simulink model "InductionMotorDrive"  (R2016a)
settings: Solver=FixedStepAuto  SolverMode=SingleTasking  StartTime=0.0  StopTime=5  FixedStep=1/400000  RelTol=1e-3
undefined symbols (not defined in the file): rad, s
libraries: powerlib x23, simulink x3, aerolibconvert2 x1, powerlib_meascontrol x1, electricdrivelib x1
settings Model: Creator=mrsmash  LastModifiedBy=mrsmash
settings SimscapeCC: SimscapeLogType=local  SimscapeLogName=simlog_Induction  SimscapeLogDataHistory=5000000

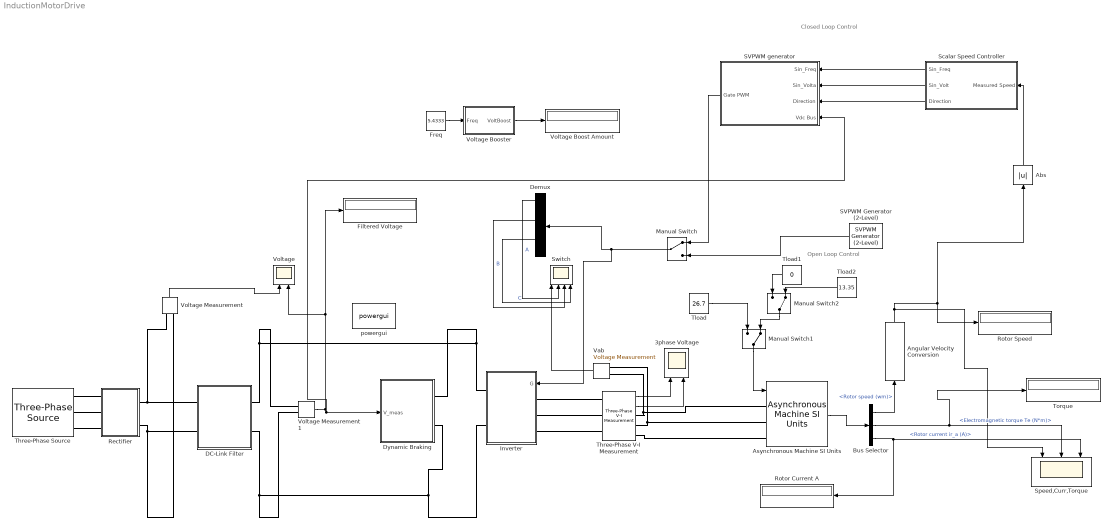
== system InductionMotorDrive ==
  note: Closed Loop Control
  note: Open Loop Control
  3phase Voltage : Scope  NumInputPorts=2
  Abs : Abs
  Angular Velocity Conversion : aerolibconvert2/Angular Velocity Conversion  IU=rad/s  OU=rpm
  Asynchronous Machine SI Units : powerlib/Machines/Asynchronous Machine SI Units  RotorType=Squirrel-cage  PresetModel=No  MechanicalLoad=Torque Tm  ShowDetailedParameters=on  ReferenceFrame=Rotor  Units=SI  MeasurementBus=off  NominalParameters=[4000 400 50]  Stator=[1.405 0.005839]  Rotor=[1.395 0.005839]  Cage1=[0.4155 0.002066]  Cage2=[0.4168 0.0003495]  Lm=0.1722  Mechanical=[0.04 0.002985 2]  PolePairs=2  InitialConditions=[1 0 0 0 0 0 0 0]  SimulateSaturation=off  Saturation=[14.03593122, 27.81365428, 53.79336849, 72.68890987, 97.98006896, 148.6815601, 215.7428561, 302.9841135, 428.7778367 ; 230, 322, 414, 460, 506, 552, 598, 644, 690]  LoadFlowParameters=1492000  TsPowergui=0  TsBlock=-1  IterativeModel=Trapezoidal non iterative  IterativeDiscreteModel=Trapezoidal non iterative  Pmec=1.492e+006
  Bus Selector : BusSelector  OutputSignals=Mechanical.Rotor speed (wm),Mechanical.Electromagnetic torque Te (N*m),Rotor measurements.Rotor current ir_a (A)
  DC-Link Filter : Subsystem
  Demux : Demux  Outputs=6
  Dynamic Braking : Subsystem
  Filtered Voltage : Display
  Freq : Constant  Value=5.4333
  Inverter : Subsystem
  Manual Switch : ManualSwitch
  Manual Switch1 : ManualSwitch  CurrentSetting=0
  Manual Switch2 : ManualSwitch  CurrentSetting=0
  Rectifier : Subsystem
  Rotor Current A : Display
  Rotor Speed : Display
  SVPWM Generator (2-Level) : powerlib_meascontrol/Pulse & Signal Generators/SVPWM Generator (2-Level)  InputType=Internally generated  SwitchingPattern=Pattern #2  Fc=10e3  ParUref=[0.1072985 0 5.43]  Ts=0
  SVPWM generator : Subsystem
  Scalar Speed Controller : Subsystem
  Speed,Curr,Torque : Scope  NumInputPorts=3
  Switch : Scope  NumInputPorts=4
  Three-Phase V-I Measurement : powerlib/Measurements/Three-Phase V-I Measurement  VoltageMeasurement=phase-to-ground  SetLabelV=off  LabelV=Vabc  Vpu=off  VpuLL=off  CurrentMeasurement=yes  SetLabelI=off  LabelI=Iabc  Ipu=off  Pbase=100e6  Vbase=500e3  OutputType=Complex  PhasorSimulation=off  PSBequivalent=0
  Three-Phase Source : powerlib/Electrical Sources/Three-Phase Source  InternalConnection=Yg  VoltagePhases=on  Voltage=25e3  PhaseAngle=0  Voltage_phases=[690 690 690]/sqrt(3)  PhaseAngles_phases=[0 -120 +120]  Frequency=50  NonIdealSource=off  SpecifyImpedance=off  Resistance=0.8929  Inductance=16.58e-3  ShortCircuitLevel=100e6  BaseVoltage=25e3  XRratio=7  BusType=swing  Pref=10e3  Qref=0  Prefabc=[10e3, 10e3, 10e3]  Qrefabc=[0, 0, 0]  Qmin=-inf  Qmax=inf
  Tload : Constant  Value=26.7
  Tload1 : Constant  Value=0
  Tload2 : Constant  Value=13.35
  Torque : Display
  Vab : powerlib/Measurements/Voltage Measurement  PhasorSimulation=off  OutputType=Complex  PSBequivalent=0
  Voltage : Scope  NumInputPorts=2
  Voltage Boost Amount : Display
  Voltage Booster : Subsystem
  Voltage Measurement : powerlib/Measurements/Voltage Measurement  PhasorSimulation=off  OutputType=Complex  PSBequivalent=0
  Voltage Measurement1 : powerlib/Measurements/Voltage Measurement  PhasorSimulation=off  OutputType=Complex  PSBequivalent=0
  powergui : powerlib/powergui  Priority=1  SimulationMode=Discrete  SolverType=Tustin/Backward Euler (TBE)  SampleTime=1/400000  frequency=60  SPID=on  DisableSnubberDevices=on  DisableRonSwitches=off  DisableVfSwitches=off  SwTol=0  DisplayEquations=off  Interpol=off  ExternalGateDelay=off  methode=off  Ts=10  FunctionMessages=off  echomessages=off  HookPort=off  EnableUseOfTLC=off  x0status=blocks  frequencyindice=50  Pbase=100e6  ErrMax=1e-4  Iterations=50  UnitsV=kV  UnitsW=MW  buscounter=0  RestoreLinks=warning  ResistiveCurrentMeasurement=off  Frange=[0:2:500]  Ylog=off  Xlog=on  ShowGrid=off  save=off  variable=ZData  structure=CurrAndVolt  ZoomFFT=off  StartTime=1.114  cycles=1  DisplayStyle=1  fundamental=50  FreqAxis=on  MaxFrequency=1500  frequencyindicesteady=1  RmsSteady=1  display=off
  wires:
  Voltage Measurement/1 -> Voltage/1
  Three-Phase V-I Measurement/1 -> 3phase Voltage/1
  Three-Phase V-I Measurement/2 -> 3phase Voltage/2
  Asynchronous Machine SI Units/1 -> Bus Selector/1
  Bus Selector/1 -> Angular Velocity Conversion/1  "<Rotor speed (wm)>"
  Bus Selector/2 -> Speed,Curr,Torque/2, Torque/1  "<Electromagnetic torque Te (N*m)>"
  Bus Selector/3 -> Speed,Curr,Torque/3, Rotor Current A/1  "<Rotor current ir_a (A)>"
  Scalar Speed Controller/2(Sin_Volt) -> SVPWM generator/2(Sin_Volta)
  SVPWM generator/1(Gate PWM) -> Manual Switch/1
  Scalar Speed Controller/3(Direction) -> SVPWM generator/3(Direction)
  Voltage Measurement1/1 -> Voltage/2, Filtered Voltage/1, SVPWM generator/4(Vdc Bus), Dynamic Braking/1(V_meas)
  SVPWM Generator (2-Level)/1 -> Manual Switch/2
  Scalar Speed Controller/1(Sin_Freq) -> SVPWM generator/1(Sin_Freq)
  Manual Switch/1 -> Inverter/1(G), Demux/1
  Demux/1 -> Switch/2  "A"
  Demux/3 -> Switch/3  "B"
  Demux/5 -> Switch/4  "C"
  Vab/1 -> Switch/1
  Manual Switch1/1 -> Asynchronous Machine SI Units/1
  Tload/1 -> Manual Switch1/1
  Angular Velocity Conversion/1 -> Speed,Curr,Torque/1, Abs/1, Rotor Speed/1
  Manual Switch2/1 -> Manual Switch1/2
  Tload2/1 -> Manual Switch2/2
  Tload1/1 -> Manual Switch2/1
  Freq/1 -> Voltage Booster/1(Freq)
  Voltage Booster/1(VoltBoost) -> Voltage Boost Amount/1
  Abs/1 -> Scalar Speed Controller/1(Measured Speed)
  connections:
  Rectifier/RConn1 -- Voltage Measurement/LConn1 -- DC-Link Filter/LConn1
  Voltage Measurement/LConn2 -- Rectifier/RConn2 -- DC-Link Filter/LConn2
  Dynamic Braking/RConn2 -- Inverter/RConn2 -- DC-Link Filter/RConn2 -- Voltage Measurement1/LConn2
  Voltage Measurement1/LConn1 -- DC-Link Filter/RConn1 -- Dynamic Braking/RConn1 -- Inverter/RConn1
  Three-Phase Source/RConn3 -- Rectifier/LConn3
  Three-Phase Source/RConn2 -- Rectifier/LConn2
  Three-Phase Source/RConn1 -- Rectifier/LConn1
  Vab/LConn2 -- Three-Phase V-I Measurement/RConn2 -- Asynchronous Machine SI Units/LConn2
  Three-Phase V-I Measurement/RConn3 -- Asynchronous Machine SI Units/LConn3
  Three-Phase V-I Measurement/RConn1 -- Asynchronous Machine SI Units/LConn1 -- Vab/LConn1
  Three-Phase V-I Measurement/LConn3 -- Inverter/LConn3
  Three-Phase V-I Measurement/LConn2 -- Inverter/LConn2
  Inverter/LConn1 -- Three-Phase V-I Measurement/LConn1

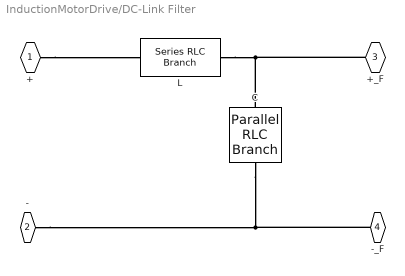
== system InductionMotorDrive/DC-Link Filter ==
  C : powerlib/Elements/Parallel RLC Branch  LConnTagsString=a  RConnTagsString=__new0  BranchType=C  Resistance=1  Inductance=1e-3  SetiL0=off  InitialCurrent=0  Capacitance=15e-3  Setx0=on  InitialVoltage=900  Measurements=None
  L : powerlib/Elements/Series RLC Branch  LConnTagsString=__new0  RConnTagsString=__new0  BranchType=L  Resistance=1  Inductance=1e-3  SetiL0=off  InitialCurrent=0  Capacitance=1e-6  Setx0=off  InitialVoltage=0  Measurements=None
  + : PMIOPort  Port=1  Side=Left
  - : PMIOPort  Port=2  Side=Left
  +_F : PMIOPort  Port=3  Side=Right
  -_F : PMIOPort  Port=4  Side=Right
  connections:
  +/RConn1 -- L/LConn1
  C/LConn1 -- L/RConn1 -- +_F/RConn1
  -/RConn1 -- C/RConn1 -- -_F/RConn1

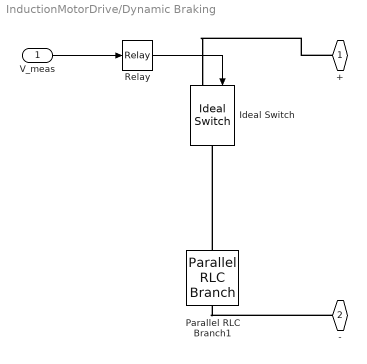
== system InductionMotorDrive/Dynamic Braking ==
  V_meas : Inport
  Ideal Switch : powerlib/Power Electronics/Ideal Switch  Ron=0.000001  Lon=0  IC=0  Rs=1e5  Cs=inf  Measurements=off
  Parallel RLC Branch1 : powerlib/Elements/Parallel RLC Branch  LConnTagsString=a  RConnTagsString=__new0  BranchType=R  Resistance=0.75  Inductance=1e-3  SetiL0=off  InitialCurrent=0  Capacitance=3.9e-3  Setx0=on  InitialVoltage=535  Measurements=None
  Relay : Relay  OnSwitchValue=1000  OffSwitchValue=900
  + : PMIOPort  Port=1  Side=Right
  - : PMIOPort  Port=2  Side=Right
  wires:
  Relay/1 -> Ideal Switch/1
  V_meas/1 -> Relay/1
  connections:
  Parallel RLC Branch1/LConn1 -- Ideal Switch/RConn1
  +/RConn1 -- Ideal Switch/LConn1
  -/RConn1 -- Parallel RLC Branch1/RConn1

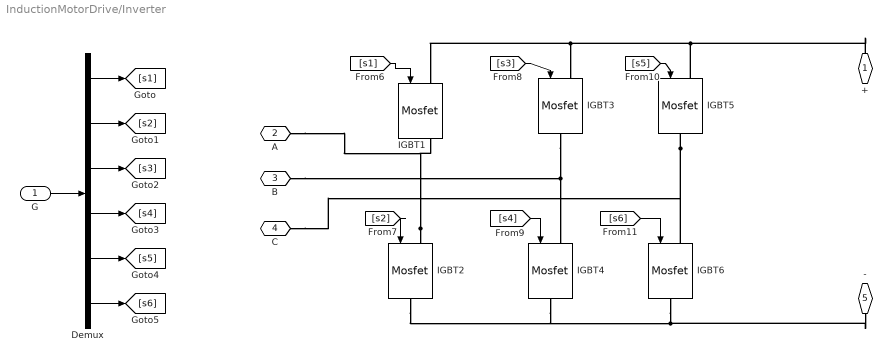
== system InductionMotorDrive/Inverter ==
  G : Inport
  Demux : Demux  Outputs=6
  IGBT1 : powerlib/Power Electronics/Mosfet  Ron=0.1  Lon=0  Rd=0.01  Vfd=0  IC=0  Rs=1e5  Cs=inf  Measurements=on
  IGBT{2..6} (5 alike) : powerlib/Power Electronics/Mosfet  Ron=0.1  Lon=0  Rd=0.01  Vfd=0  IC=0  Rs=1e5  Cs=inf  Measurements=off
  + : PMIOPort  Port=1  Side=Right
  A : PMIOPort  Port=2  Side=Left
  B : PMIOPort  Port=3  Side=Left
  C : PMIOPort  Port=4  Side=Left
  - : PMIOPort  Port=5  Side=Right
  wires:
  [s1] -> IGBT1/1
  [s2] -> IGBT2/1
  [s3] -> IGBT3/1
  [s4] -> IGBT4/1
  [s5] -> IGBT5/1
  [s6] -> IGBT6/1
  Demux/1 -> [s1]
  Demux/2 -> [s2]
  Demux/3 -> [s3]
  Demux/4 -> [s4]
  Demux/5 -> [s5]
  Demux/6 -> [s6]
  G/1 -> Demux/1
  connections:
  IGBT5/LConn1 -- IGBT1/LConn1 -- IGBT3/LConn1 -- +/RConn1
  IGBT6/RConn1 -- -/RConn1 -- IGBT2/RConn1 -- IGBT4/RConn1
  IGBT2/LConn1 -- IGBT1/RConn1 -- A/RConn1
  IGBT3/RConn1 -- IGBT4/LConn1 -- B/RConn1
  IGBT5/RConn1 -- IGBT6/LConn1 -- C/RConn1

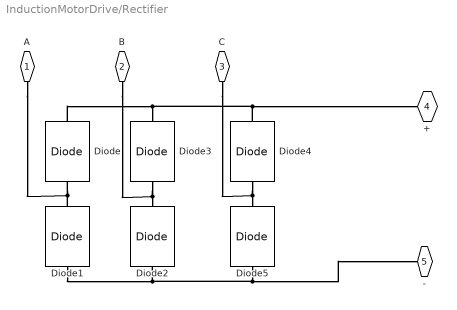
== system InductionMotorDrive/Rectifier ==
  Diode{,1..5} (6 alike) : powerlib/Power Electronics/Diode  Ron=0.001  Lon=0  Vf=0.8  IC=0  UseSnubber=off  Rs=500  Cs=250e-9  Measurements=off
  A : PMIOPort  Port=1  Side=Left
  B : PMIOPort  Port=2  Side=Left
  C : PMIOPort  Port=3  Side=Left
  + : PMIOPort  Port=4  Side=Right
  - : PMIOPort  Port=5  Side=Right
  connections:
  Diode/LConn1 -- A/RConn1 -- Diode1/RConn1
  Diode5/RConn1 -- C/RConn1 -- Diode4/LConn1
  Diode3/RConn1 -- +/RConn1 -- Diode4/RConn1 -- Diode/RConn1
  Diode2/RConn1 -- B/RConn1 -- Diode3/LConn1
  Diode5/LConn1 -- -/RConn1 -- Diode1/LConn1 -- Diode2/LConn1

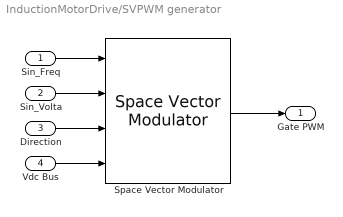
== system InductionMotorDrive/SVPWM generator ==
  Sin_Freq : Inport
  Sin_Volta : Inport  Port=2
  Direction : Inport  Port=3
  Vdc Bus : Inport  Port=4
  Space Vector Modulator : electricdrivelib/Fundamental Drive Blocks/Space Vector Modulator  OverrideUsingVariant=Detailed  detailLevel=Detailed  fc_bus=50  car_freq=10e3  TsMLIV=20e-6  Ts=2.5e-6
      settings: AttributesFormatString=%<BlockChoice>
  Gate PWM : Outport
  wires:
  Sin_Freq/1 -> Space Vector Modulator/1
  Sin_Volta/1 -> Space Vector Modulator/2
  Direction/1 -> Space Vector Modulator/3
  Space Vector Modulator/1 -> Gate PWM/1
  Vdc Bus/1 -> Space Vector Modulator/4

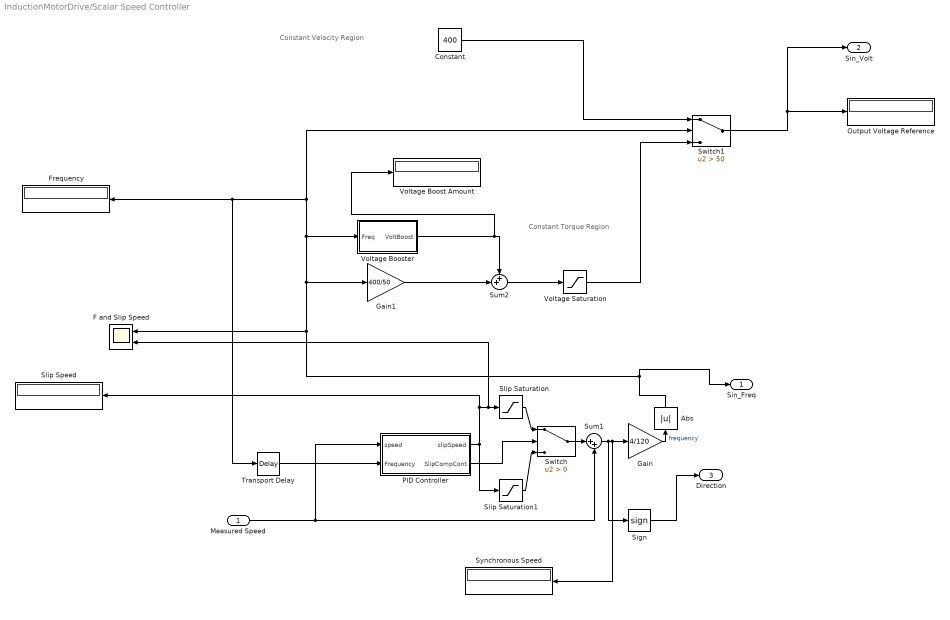
== system InductionMotorDrive/Scalar Speed Controller ==
  note: Constant Torque Region
  note: Constant Velocity Region
  Measured Speed : Inport
  Abs : Abs
  Constant : Constant  Value=400
  F and Slip Speed : Scope  NumInputPorts=2
  Frequency : Display
  Gain : Gain  Gain=4/120
  Gain1 : Gain  Gain=400/50
  Output Voltage Reference : Display
  PID Controller : Subsystem
  Sign : Signum
  Slip Saturation : Saturate  UpperLimit=1000  LowerLimit=-1000
  Slip Saturation1 : Saturate  UpperLimit=100  LowerLimit=-100
  Slip Speed : Display
  Sum1 : Sum  Inputs=|++
  Sum2 : Sum  Inputs=++|
  Switch : Switch  Criteria=u2 > Threshold
  Switch1 : Switch  Criteria=u2 > Threshold  Threshold=50
  Synchronous Speed : Display
  Transport Delay : TransportDelay  DelayTime=1/200000
  Voltage Boost Amount : Display
  Voltage Booster : Subsystem
  Voltage Saturation : Saturate  UpperLimit=400*1.5  LowerLimit=-100
  Sin_Freq : Outport
  Sin_Volt : Outport  Port=2
  Direction : Outport  Port=3
  wires:
  Sum1/1 -> Sign/1, Synchronous Speed/1, Gain/1
  Gain/1 -> Abs/1  "frequency"
  Measured Speed/1 -> Sum1/2, PID Controller/1(speed)
  Voltage Booster/1(VoltBoost) -> Sum2/1, Voltage Boost Amount/1
  Sum2/1 -> Voltage Saturation/1
  Sign/1 -> Direction/1
  Switch/1 -> Sum1/1
  Slip Saturation/1 -> Switch/1
  Slip Saturation1/1 -> Switch/3
  PID Controller/1(slipSpeed) -> Slip Saturation1/1, Slip Speed/1, F and Slip Speed/2, Slip Saturation/1
  PID Controller/2(SlipCompCont) -> Switch/2
  Switch1/1 -> Sin_Volt/1, Output Voltage Reference/1
  Gain1/1 -> Sum2/2
  Constant/1 -> Switch1/1
  Voltage Saturation/1 -> Switch1/3
  Transport Delay/1 -> PID Controller/2(Frequency)
  Abs/1 -> Sin_Freq/1, F and Slip Speed/1, Voltage Booster/1(Freq), Transport Delay/1, Frequency/1, Switch1/2, Gain1/1

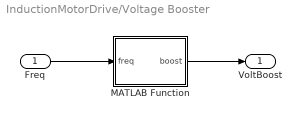
== system InductionMotorDrive/Voltage Booster ==
  Freq : Inport
  MATLAB Function : MATLAB Function  TreatAsAtomicUnit=on
  VoltBoost : Outport
  wires:
  Freq/1 -> MATLAB Function/1(freq)
  MATLAB Function/1(boost) -> VoltBoost/1

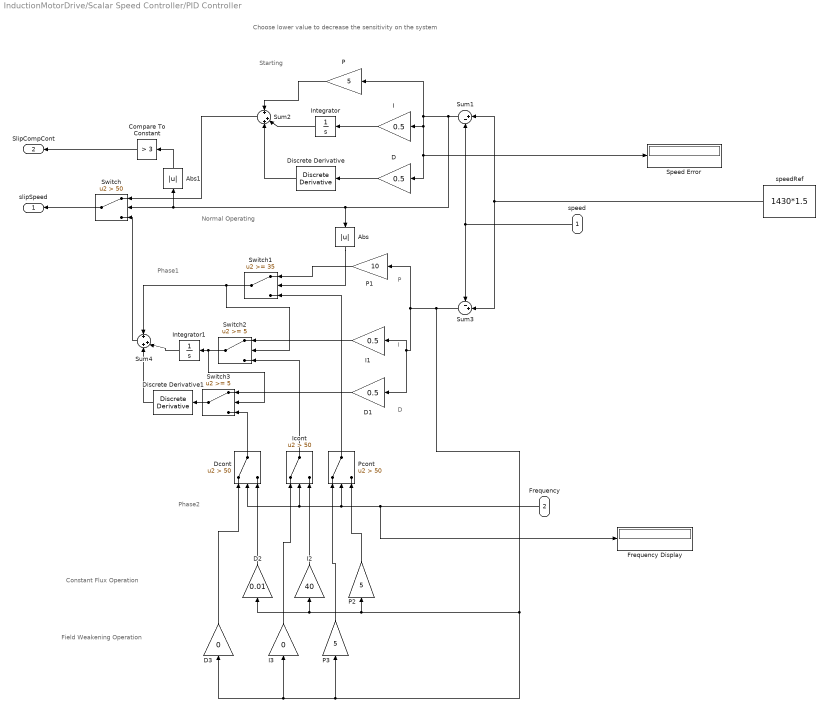
== system InductionMotorDrive/Scalar Speed Controller/PID Controller ==
  note: P
  note: Phase1
  note: Normal Operating
  note: Starting
  note: Choose lower value to decrease the sensitivity on the system
  note: Phase2
  note: I
  note: D
  note: Field Weakening Operation
  note: Constant Flux Operation
  speed : Inport
  Frequency : Inport  Port=2
  Abs : Abs
  Abs1 : Abs
  Compare To Constant : simulink/Logic and Bit Operations/Compare To Constant  relop=>  const=3  OutDataTypeStr=boolean
  D : Gain  Gain=0.5
  D1 : Gain  Gain=0.5
  D2 : Gain  Gain=0.01
  D3 : Gain  Gain=0
  Dcont : Switch  Criteria=u2 > Threshold  Threshold=50
  Discrete Derivative : simulink/Discrete/Discrete Derivative  gainval=1.0  ICPrevScaledInput=0.0  OutMin=[]  OutMax=[]  OutDataType=fixdt(1, 16)  OutScaling=2^-10  DoSatur=off
  Discrete Derivative1 : simulink/Discrete/Discrete Derivative  gainval=1.0  ICPrevScaledInput=0.0  OutMin=[]  OutMax=[]  OutDataType=fixdt(1, 16)  OutScaling=2^-10  DoSatur=off
  Frequency Display : Display
  I : Gain  Gain=0.5
  I1 : Gain  Gain=0.5
  I2 : Gain  Gain=40
  I3 : Gain  Gain=0
  Icont : Switch  Criteria=u2 > Threshold  Threshold=50
  Integrator : Integrator
  Integrator1 : Integrator
  P : Gain  Gain=5
  P1 : Gain  Gain=10
  P2 : Gain  Gain=5
  P3 : Gain  Gain=5
  Pcont : Switch  Criteria=u2 > Threshold  Threshold=50
  Speed Error : Display
  Sum1 : Sum  Inputs=|+-
  Sum2 : Sum  Inputs=+|++
  Sum3 : Sum  Inputs=-+|
  Sum4 : Sum  Inputs=+|++
  Switch : Switch  Criteria=u2 > Threshold  Threshold=50
  Switch1 : Switch  Threshold=35
  Switch2 : Switch  Threshold=5
  Switch3 : Switch  Threshold=5
  speedRef : Constant  Value=1430*1.5  SampleTime=-1
  slipSpeed : Outport
  SlipCompCont : Outport  Port=2
  wires:
  P/1 -> Sum2/1
  I/1 -> Integrator/1
  Integrator/1 -> Sum2/2
  D/1 -> Discrete Derivative/1
  Discrete Derivative/1 -> Sum2/3
  Switch1/1 -> Switch2/2, Sum4/1
  Integrator1/1 -> Sum4/2
  Discrete Derivative1/1 -> Sum4/3
  speedRef/1 -> Sum3/2, Sum1/1
  Sum1/1 -> Abs/1, Switch/2, Abs1/1, P/1, D/1, Speed Error/1, I/1
  Sum2/1 -> Switch/1
  Compare To Constant/1 -> SlipCompCont/1
  Sum4/1 -> Switch/3
  P1/1 -> Switch1/1
  Pcont/1 -> Switch1/3
  I1/1 -> Switch2/1
  Icont/1 -> Switch2/3
  Switch2/1 -> Switch3/2, Integrator1/1
  Switch3/1 -> Discrete Derivative1/1
  D1/1 -> Switch3/1
  Dcont/1 -> Switch3/3
  Abs/1 -> Switch1/2
  Switch/1 -> slipSpeed/1
  Sum3/1 -> D2/1, I2/1, P2/1, D3/1, I3/1, P3/1, D1/1, I1/1, P1/1
  Frequency/1 -> Frequency Display/1, Dcont/2, Icont/2, Pcont/2
  D2/1 -> Dcont/3
  I2/1 -> Icont/3
  P2/1 -> Pcont/3
  P3/1 -> Pcont/1
  I3/1 -> Icont/1
  D3/1 -> Dcont/1
  Abs1/1 -> Compare To Constant/1
  speed/1 -> Sum3/1, Sum1/2

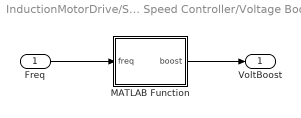
== system InductionMotorDrive/Scalar Speed Controller/Voltage Booster ==
  Freq : Inport
  MATLAB Function : MATLAB Function  TreatAsAtomicUnit=on
  VoltBoost : Outport
  wires:
  Freq/1 -> MATLAB Function/1(freq)
  MATLAB Function/1(boost) -> VoltBoost/1

== matlab function InductionMotorDrive/Voltage Booster/MATLAB Function ==
  data: freq input; boost output
function boost = fcn(freq)
    boost = 0 ;
    %Voltage Boost Calculator
    
    TMax = 91.0303 ; %Max Torque

    Ls = 5.839e-3 ; %Stator Inductance Henry
    Lm = 0.1722 ; % Magnetization Inductance Henry
    Lr = 5.839e-3 ; % Rotor inductance Henry
    Rs = 1.405 ; % Stator resistance ohm
    
    VRated = 230 ; 
    frated = 50 ;
    p =4 ;
    if (freq ~= 0) && (freq < 50) 
        constant = 50/freq;
        fRated = frated/constant;

        ws = 2*pi*fRated/(p/2);

        Xs = Ls*2*pi*fRated ; 
        Xr = Lr*2*pi*fRated;
        Xm = Lm*2*pi*fRated;

        Zth = (-Xm*Xs+1i*Rs*Xm)/(Rs+1i*(Xs+Xm));
        Rth = real(Zth);
        Xth = imag(Zth);

        %To find how much voltage we have to boost,I used our maximum torque value 
        %So I derived needed thevenin voltage for current frequency
        Vboost_1 = sqrt(complex(TMax*(2*ws*(Rth+sqrt(Rth^2+(Xth+Xr)^2)))/3));
        Vboost_2 = Vboost_1*(Rs+1i*(Xs+Xm))/(1i*Xm)-VRated/constant;

        boost= real(Vboost_2);
    else
        return
    end
end

== matlab function InductionMotorDrive/Scalar Speed Controller/Voltage Booster/MATLAB Function ==
  data: freq input; boost output
function boost = fcn(freq)
    boost = 0 ;
    %Voltage Boost Calculator
    
    TMax = 91.0303 ; %Max Torque

    Ls = 5.839e-3 ; %Stator Inductance Henry
    Lm = 0.1722 ; % Magnetization Inductance Henry
    Lr = 5.839e-3 ; % Rotor inductance Henry
    Rs = 1.405 ; % Stator resistance ohm
    
    VRated = 230 ; 
    frated = 50 ;
    p =4 ;
    if (freq ~= 0) && (freq < 50) 
        constant = 50/freq;
        fRated = frated/constant;

        ws = 2*pi*fRated/(p/2);

        Xs = Ls*2*pi*fRated ; 
        Xr = Lr*2*pi*fRated;
        Xm = Lm*2*pi*fRated;

        Zth = (-Xm*Xs+1i*Rs*Xm)/(Rs+1i*(Xs+Xm));
        Rth = real(Zth);
        Xth = imag(Zth);

        %To find how much voltage we have to boost,I used our maximum torque value 
        %So I derived needed thevenin voltage for current frequency
        Vboost_1 = sqrt(complex(TMax*(2*ws*(Rth+sqrt(Rth^2+(Xth+Xr)^2)))/3));
        Vboost_2 = Vboost_1*(Rs+1i*(Xs+Xm))/(1i*Xm)-VRated/constant;

        boost= real(Vboost_2);
    else
        return
    end
end
